simulink model "Bouncing"  (R2022a)
settings: Solver=FixedStepAuto  StartTime=0.0  StopTime=25  FixedStep=0.01  RelTol=1e-3
model workspace (MAT data in the model file):
  slope = 0
settings Model: Creator=黃冠融  LastModifiedBy=黃冠融

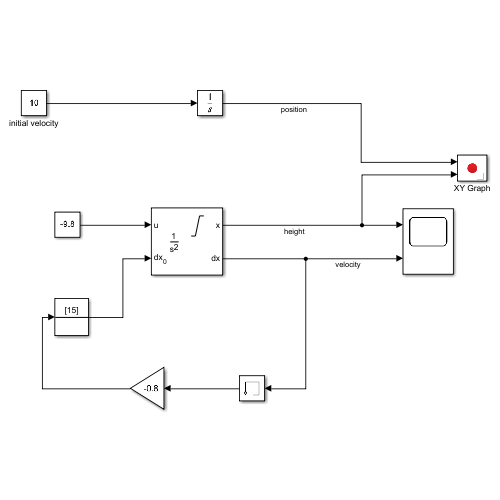
[thumbnail: Simulink's stored preview of the top-level diagram]
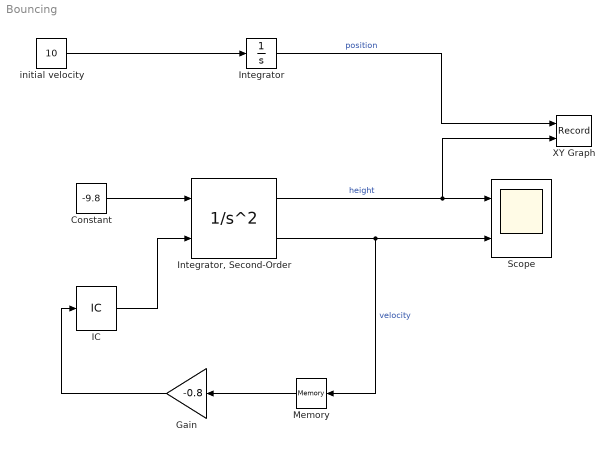
== system Bouncing ==
  Constant : Constant  Value=-9.8
  Gain : Gain  Gain=-0.8
  IC : InitialCondition  Value=15
  Integrator : Integrator
  "Integrator, Second-Order" : SecondOrderIntegrator  ICX=10  LimitX=on  LowerLimitX=slope  StateNameX=Position  ICSourceDXDT=external  StateNameDXDT=Velocity  ReinitDXDTwhenXreachesSaturation=on
  Memory : Memory
  Scope : Scope  NumInputPorts=2
  XY Graph : Record  FileSettingsInternal="{\"entries\":[{\"content\":{\"excelSettings\":{\"content\":{},\"type\":\"Streamout.ExcelSettings\"}},\"type\":\"Streamout.FileSettingStorage\",\"uuid\":\"5cd439fa-0efb-4231-93b2-fedac9df6622\"}],\"packageUris\":[\"http://schema.mathworks.com/mf0/streamout_blocks/R2020a\"],\"version\":\"1.0\"}"  Layout=[1 1]  SignalsInternal="{\"entries\":[{\"content\":{\"signals\":[{\"content\":{\"blockPath\":[\"Bouncing/XY Graph\"],\"channel\":[],\"dimensions\":[1],\"domain\":\"Bouncing/XY Graph\",\"lineColor\":\"#a2142f\",\"plots\":[1],\"port\":1,\"sid\":[\"\"],\"signalID\":194,\"signalName\":\"position\"},\"type\":\"RecordBlkView.Signal\",\"uuid\":\"b6e03530-ed83-44cf-8459-a96219ff4139\"},{\"content\":{\"blockPath\":[\"Bouncing/XY Graph\"],\"channel\":[],\"dimensions\":[1],\"domain\":\"Bouncing/XY Graph\",\"lineColor\":\"#139fff\",\"plots\":[1],\"port\":2,\"sid\":[\"\"],\"signalID\":198,\"signalName\":\"height\"},\"type\":\"RecordBlkView.Signal\",\"uuid\":\"48b4f498-a151-4686-affc-f143031f2b74\"}]},\"type\":\"RecordBlkView.InputSignals\",\"uuid\":\"c02f89fe-45ce-4a09-ab86-37144a34c205\"}],\"packageUris\":[\"http://schema.mathworks.com/mf0/streamout_blocks/R2020a\"],\"version\":\"1.0\"}"  VisualizationBindings="{\"xyplotplugin\":{\"info\":[{\"series\":[{\"bindingParametersList\":[{\"parameter\":\"X-Axis\",\"signalID\":194,\"signalName\":\"position\"},{\"parameter\":\"Y-Axis\",\"signalID\":198,\"signalName\":\"height\"}],\"seriesID\":25449}],\"subplotID\":1}]}}"  CompatibilityTag=XY
  initial velocity : Constant  Value=10
  wires:
  "Integrator, Second-Order"/2 -> Memory/1, Scope/2  "velocity"
  "Integrator, Second-Order"/1 -> XY Graph/2, Scope/1  "height"
  Memory/1 -> Gain/1
  Gain/1 -> IC/1
  IC/1 -> "Integrator, Second-Order"/2
  Constant/1 -> "Integrator, Second-Order"/1
  initial velocity/1 -> Integrator/1
  Integrator/1 -> XY Graph/1  "position"
